simulink model "ThrustModel_LIM"  (R2020a)
settings: Solver=VariableStepAuto  StartTime=0.0  StopTime=10.0  RelTol=1e-3
settings Model: Creator=James Bates  LastModifiedBy=James Bates

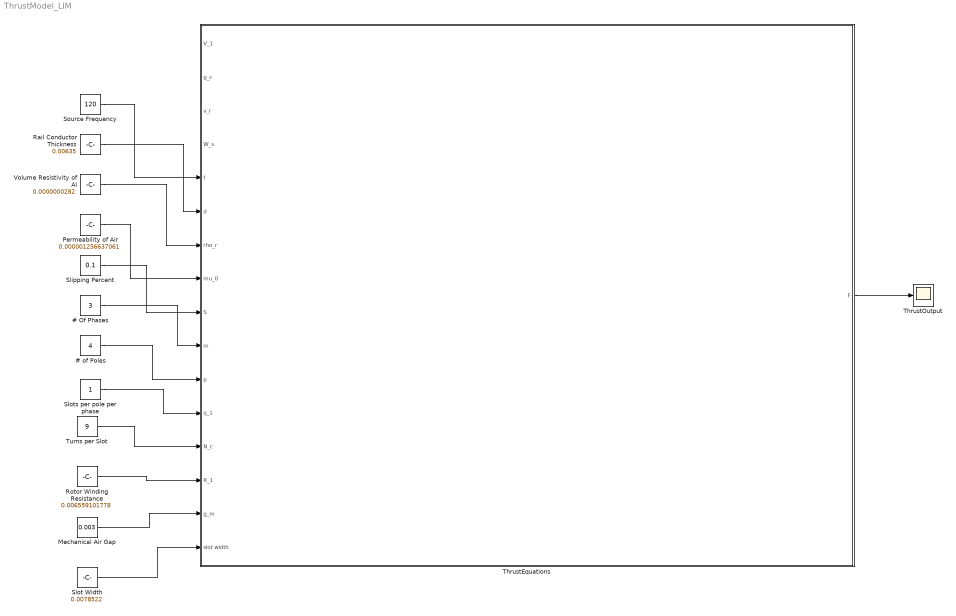
== system ThrustModel_LIM ==
  # Of Phases : Constant  Value=3
  # of Poles : Constant  Value=4
  Mechanical Air Gap : Constant  Value=0.003
  Permeability of Air : Constant  Value=0.000001256637061
  Rail Conductor Thickness : Constant  Value=0.00635
  Rotor Winding Resistance : Constant  Value=0.006559101778
  Slipping Percent : Constant  Value=0.1
  Slot Width : Constant  Value=0.0078522
  Slots per pole per phase : Constant
  Source Frequency : Constant  Value=120
  ThrustEquations : Subsystem
  ThrustOutput : Scope
  Turns per Slot : Constant  Value=9
  Volume Resistivity of Al : Constant  Value=0.0000000282
  wires:
  ThrustEquations/1(F) -> ThrustOutput/1
  Source Frequency/1 -> ThrustEquations/5(f)
  Rail Conductor Thickness/1 -> ThrustEquations/6(d)
  Volume Resistivity of Al/1 -> ThrustEquations/7(rho_r)
  Permeability of Air/1 -> ThrustEquations/8(mu_0)
  Slipping Percent/1 -> ThrustEquations/9(S)
  # Of Phases/1 -> ThrustEquations/10(m)
  Slots per pole per phase/1 -> ThrustEquations/12(q_1)
  # of Poles/1 -> ThrustEquations/11(p)
  Turns per Slot/1 -> ThrustEquations/13(N_c)
  Rotor Winding Resistance/1 -> ThrustEquations/14(R_1)
  Mechanical Air Gap/1 -> ThrustEquations/15(g_m)
  Slot Width/1 -> ThrustEquations/16(slot width)

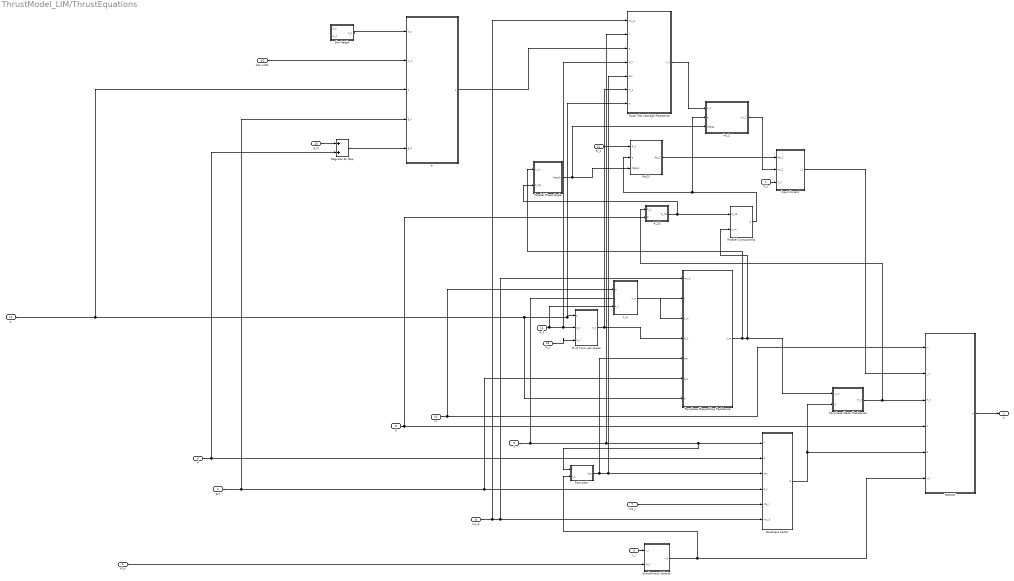
== system ThrustModel_LIM/ThrustEquations ==
  V_1 : Inport
  g_c : Inport  Port=2
  v_r : Inport  Port=3
  W_s : Inport  Port=4
  f : Inport  Port=5
  d : Inport  Port=6
  rho_r : Inport  Port=7
  mu_0 : Inport  Port=8
  S : Inport  Port=9
  m : Inport  Port=10
  p : Inport  Port=11
  q_1 : Inport  Port=12
  N_c : Inport  Port=13
  R_1 : Inport  Port=14
  g_m : Inport  Port=15
  slot width : Inport  Port=16
  " Input Current" : MATLAB Function  TreatAsAtomicUnit=on
  # of Turns per phase : MATLAB Function  TreatAsAtomicUnit=on
  Goodness Factor : MATLAB Function  TreatAsAtomicUnit=on
  Magnetic Air Gap : Sum
  Parallel Components : MATLAB Function  TreatAsAtomicUnit=on
  Parallel Phase Angle : MATLAB Function  TreatAsAtomicUnit=on
  Per-phase Magnetizing Resistance : MATLAB Function  TreatAsAtomicUnit=on
  "Per-phase Stator Resistance " : MATLAB Function  TreatAsAtomicUnit=on
  Pole pitch : MATLAB Function  TreatAsAtomicUnit=on
  R_2S : MATLAB Function  TreatAsAtomicUnit=on
  Re(Z) : MATLAB Function  TreatAsAtomicUnit=on
  Rotor Slot Leakage Reactance : MATLAB Function  TreatAsAtomicUnit=on
  Slot Height : MATLAB Function  TreatAsAtomicUnit=on
  Synchronous Velocity : MATLAB Function  TreatAsAtomicUnit=on
  THRUST : MATLAB Function  TreatAsAtomicUnit=on
  a : MATLAB Function  TreatAsAtomicUnit=on
  k_w : MATLAB Function  TreatAsAtomicUnit=on
  lm_Z : MATLAB Function  TreatAsAtomicUnit=on
  F : Outport
  wires:
  "Per-phase Stator Resistance "/1(R_2) -> R_2S/1(R_2), THRUST/3(R_2)
  Goodness Factor/1(G) -> "Per-phase Stator Resistance "/2(G), THRUST/5(G)
  f/1 -> Per-phase Magnetizing Resistance/2(f), Rotor Slot Leakage Reactance/2(f), Pole pitch/1(f), Goodness Factor/1(f)
  m/1 -> k_w/1(m), THRUST/1(m)
  Synchronous Velocity/1(v_s) -> Pole pitch/2(v_s), THRUST/6(v_s)
  mu_0/1 -> Rotor Slot Leakage Reactance/1(mu_0), Per-phase Magnetizing Resistance/1(mu_0), Goodness Factor/6(mu_0)
  rho_r/1 -> Goodness Factor/5(rho_r)
  S/1 -> R_2S/2(S), THRUST/4(S)
  Pole pitch/1(tau) -> Per-phase Magnetizing Resistance/5(tau), Rotor Slot Leakage Reactance/5(tau), Goodness Factor/3(tau)
  " Input Current"/1(I_1) -> THRUST/2(I_1)
  d/1 -> Magnetic Air Gap/2, Goodness Factor/2(d)
  V_1/1 -> " Input Current"/3(V_1)
  W_s/1 -> Synchronous Velocity/2(W_s)
  v_r/1 -> Synchronous Velocity/1(v_r)
  g_c/1 -> a/4(g_c), Per-phase Magnetizing Resistance/6(g_c), Goodness Factor/4(g_c)
  THRUST/1(F) -> F/1
  Per-phase Magnetizing Resistance/1(X_m) -> Parallel Phase Angle/1(X_m), Parallel Components/2(X_m), "Per-phase Stator Resistance "/1(X_m)
  # of Turns per phase/1(N_1) -> Rotor Slot Leakage Reactance/6(N_1), Per-phase Magnetizing Resistance/4(N_1)
  p/1 -> a/3(p), Per-phase Magnetizing Resistance/7(p), Rotor Slot Leakage Reactance/7(p), # of Turns per phase/1(p)
  q_1/1 -> k_w/2(q_1), Rotor Slot Leakage Reactance/4(q_1), # of Turns per phase/2(q_1)
  N_c/1 -> # of Turns per phase/3(N_c)
  k_w/1(k_w) -> Per-phase Magnetizing Resistance/3(k_w)
  Re(Z)/1(Re_Z) -> " Input Current"/1(Re_Z)
  R_1/1 -> Re(Z)/1(R_1)
  Parallel Components/1(b) -> lm_Z/2(b), Re(Z)/2(b)
  R_2S/1(R_2S) -> Parallel Phase Angle/2(R_2S), Parallel Components/1(R_2S)
  Parallel Phase Angle/1(theta2) -> lm_Z/3(theta2), Re(Z)/3(theta2)
  lm_Z/1(lm_Z) -> " Input Current"/2(Im_Z)
  Rotor Slot Leakage Reactance/1(X_1) -> lm_Z/1(X_1)
  a/1(a) -> Rotor Slot Leakage Reactance/3(a)
  Magnetic Air Gap/1 -> a/5(g_0)
  g_m/1 -> Magnetic Air Gap/1
  slot width/1 -> a/2(w_s)
  Slot Height/1(h_s) -> a/1(h_s)

== matlab function ThrustModel_LIM/ThrustEquations/Re(Z) ==
  data: R_1 input; Re_Z output; b input; theta2 input
function Re_Z = fcn(R_1, b, theta2)

Re_Z = R_1+b*cos(theta2);

== matlab function ThrustModel_LIM/ThrustEquations/Parallel Components ==
  data: R_2S input; b output; X_m input
function b = fcn(R_2S, X_m)

b = (R_2S*X_m)/sqrt(X_m*X_m+R_2S*R_2S);

== matlab function ThrustModel_LIM/ThrustEquations/R_2S ==
  data: R_2 input; R_2S output; S input
function R_2S = fcn(R_2, S)

R_2S = R_2 / S;

== matlab function ThrustModel_LIM/ThrustEquations/Parallel Phase Angle ==
  data: X_m input; theta2 output; R_2S input
function theta2 = fcn(X_m, R_2S)

theta2 = pi/2-atan(X_m/R_2S);

== matlab function ThrustModel_LIM/ThrustEquations/Goodness Factor ==
  data: f input; G output; d input; tau input; g_c input; rho_r input; mu_0 input
function G = fcn(f,d,tau,g_c,rho_r,mu_0)
%f & d are Variables
% mu_0 is a Constant
G = 2*mu_0*f*tau*tau/(pi*g_c*(rho_r/d));

== matlab function ThrustModel_LIM/ThrustEquations/lm_Z ==
  data: X_1 input; lm_Z output; b input; theta2 input
function lm_Z = fcn(X_1, b, theta2)

lm_Z = X_1+b*sin(theta2);

== matlab function ThrustModel_LIM/ThrustEquations/Rotor Slot Leakage Reactance ==
  data: mu_0 input; X_1 output; f input; a input; q_1 input; tau input; N_1 input; p input
function X_1 = fcn(mu_0, f, a, q_1, tau, N_1, p)

X_1 = 8*mu_0*pi*f*((a*pi)/q_1+0.6*tau)*N_1*N_1/p;

== matlab function ThrustModel_LIM/ThrustEquations/a ==
  data: h_s input; a output; w_s input; p input; g_c input; g_0 input
function a = fcn(h_s, w_s, p, g_c, g_0)

a = (h_s/(3*w_s))*(1+3/p)+5*(g_c/w_s)/(5+4*(g_0/w_s));

== matlab function ThrustModel_LIM/ThrustEquations/Slot Height ==
  data: A_s input; h_s output; w_s input
function h_s = fcn(A_s, w_s)

h_s = A_s/w_s;

== matlab function ThrustModel_LIM/ThrustEquations/THRUST ==
  data: m input; F output; I_1 input; R_2 input; S input; G input; v_s input
function F = fcn(m,I_1,R_2,S,G,v_s)

F = m*(I_1*I_1)*R_2/((1/(S*S*G*G)+1)*S*v_s);

== matlab function ThrustModel_LIM/ThrustEquations/Synchronous Velocity ==
  data: v_r input; v_s output; W_s input
function v_s = fcn(v_r, W_s)
% Both inputs are variables

v_s = v_r/(1-W_s);

== matlab function ThrustModel_LIM/ThrustEquations/Per-phase Stator Resistance  ==
  data: X_m input; R_2 output; G input
function R_2 = fcn(X_m, G)

R_2 = X_m/G;

== matlab function ThrustModel_LIM/ThrustEquations/ Input Current ==
  data: Re_Z input; I_1 output; Im_Z input; V_1 input
function I_1 = fcn(Re_Z, Im_Z, V_1)
%Re_Z = Re(Z)
%Im_Z = Im(Z)

I_1 = V_1/sqrt(Re_Z*Re_Z+Im_Z*Im_Z);

== matlab function ThrustModel_LIM/ThrustEquations/Pole pitch ==
  data: f input; tau output; v_s input
function tau = fcn(f, v_s)

tau = v_s/(2*f);

== matlab function ThrustModel_LIM/ThrustEquations/Per-phase Magnetizing Resistance ==
  data: mu_0 input; X_m output; f input; k_w input; N_1 input; tau input; g_c input; p input
function X_m = fcn(mu_0, f, k_w, N_1, tau, g_c, p)

X_m = 24*mu_0*pi*f*k_w*N_1*N_1*tau(pi+g_c)/(pi*pi*p*g_c);

== matlab function ThrustModel_LIM/ThrustEquations/# of Turns per phase ==
  data: p input; N_1 output; q_1 input; N_c input
function N_1 = fcn(p, q_1, N_c)

N_1 = p*q_1*N_c;

== matlab function ThrustModel_LIM/ThrustEquations/k_w ==
  data: m input; k_w output; q_1 input
function k_w = fcn(m, q_1)

k_w = sin(pi/(2*m))/(q_1*sin(pi/(2*m*q_1)));
